simulink model "linModel_S_LQG"  (R2021b)
settings: Solver=ode45  StartTime=0.0  StopTime=0.5  MaxStep=0.01  RelTol=1e-8
values from neighbouring files (symbols this model uses):
  A = [0 1; -k/mass-(4*C_magnetic*Ib^2)/(mass*gap^3) -c/mass]    [ex4.m]    (also in mp62.m = [-2 -3;-1 -4]; od.m = [0 1; -k/m-(4*C_magnetic*Ib^2)/(m*gap^3) -c/m])
  B = [0;(4*C_magnetic*Ib)/(mass*gap^2)]    [ex4.m]    (also in mp62.m = [0 1]'; od.m = [0;(4*C_magnetic*Ib)/(m*gap^2)])
  C = 0.0157    [ex2_1.m]    (also in ex3.m = 3.73e-06; ex4.m = [1 0]; mp62.m = [1 0]; od.m = [1 0;0 0])
  D = 0    [ex4.m]    (also in mp62.m; od.m)
  Kf = lqr(A',C',Vd,Vn)    [ex4.m]
  L = acker(A',C',P)'    [mp62.m]
undefined symbols (not defined in the file or in its folder): Kr
settings Model: Creator=danli  LastModifiedBy=danli

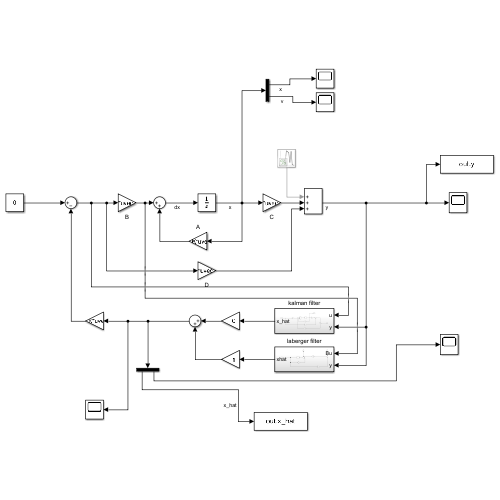
[thumbnail: Simulink's stored preview of the top-level diagram]
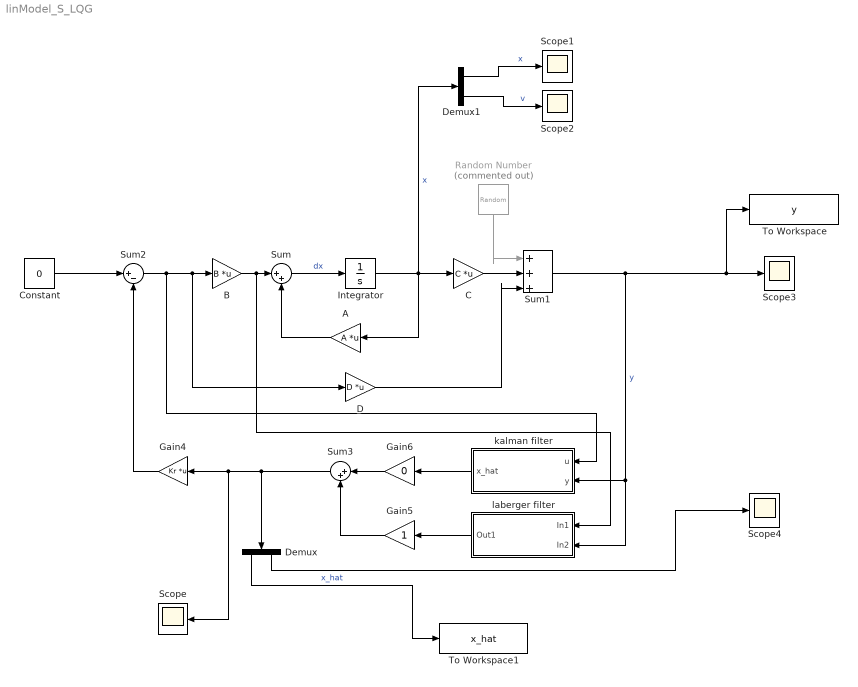
== system linModel_S_LQG ==
  A : Gain  Gain=A  Multiplication=Matrix(K*u) (u vector)
  B : Gain  Gain=B  Multiplication=Matrix(K*u) (u vector)
  C : Gain  Gain=C  Multiplication=Matrix(K*u) (u vector)
  Constant : Constant  Value=0
  D : Gain  Gain=D  Multiplication=Matrix(K*u) (u vector)
  Demux : Demux  Outputs=2
  Demux1 : Demux  Outputs=2
  Gain4 : Gain  Gain=Kr  Multiplication=Matrix(K*u) (u vector)
  Gain5 : Gain
  Gain6 : Gain  Gain=0
  Integrator : Integrator  InitialCondition=[5*10^-5 0]
  Random Number : RandomNumber  Commented=on  Variance=0.0000000000001  SampleTime=0.001
  Scope{,1..4} (5 alike) : Scope
  Sum : Sum  Inputs=|++
  Sum1 : Sum  Inputs=|+|+|+
  Sum2 : Sum  Inputs=|+-
  Sum3 : Sum  Inputs=|++
  To Workspace : ToWorkspace  VariableName=y  SaveFormat=Timeseries  SampleTime=-1
  To Workspace1 : ToWorkspace  VariableName=x_hat  SaveFormat=Timeseries  SampleTime=-1
  kalman filter : Subsystem
  laberger filter : Subsystem
  wires:
  B/1 -> laberger filter/1(In1), Sum/1
  A/1 -> Sum/2
  Sum/1 -> Integrator/1  "dx"
  Integrator/1 -> A/1, Demux1/1, C/1  "x"
  D/1 -> Sum1/3
  C/1 -> Sum1/2
  Sum2/1 -> kalman filter/1(u), D/1, B/1
  Constant/1 -> Sum2/1
  Gain4/1 -> Sum2/2
  Demux1/1 -> Scope1/1  "x"
  Demux1/2 -> Scope2/1  "v"
  Sum1/1 -> To Workspace/1, Scope3/1, laberger filter/2(In2), kalman filter/2(y)  "y"
  Random Number/1 -> Sum1/1
  Demux/1 -> To Workspace1/1  "x_hat"
  Demux/2 -> Scope4/1
  laberger filter/1(Out1) -> Gain5/1
  Gain5/1 -> Sum3/2
  kalman filter/1(x_hat) -> Gain6/1
  Gain6/1 -> Sum3/1
  Sum3/1 -> Demux/1, Scope/1, Gain4/1

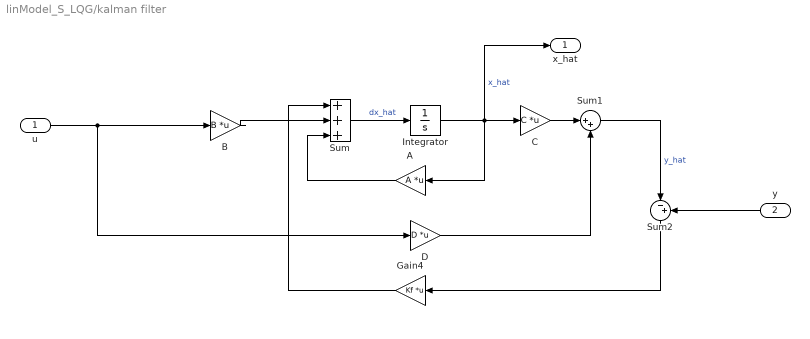
== system linModel_S_LQG/kalman filter ==
  u : Inport
  y : Inport  Port=2
  A : Gain  Gain=A  Multiplication=Matrix(K*u) (u vector)
  B : Gain  Gain=B  Multiplication=Matrix(K*u) (u vector)
  C : Gain  Gain=C  Multiplication=Matrix(K*u) (u vector)
  D : Gain  Gain=D  Multiplication=Matrix(K*u) (u vector)
  Gain4 : Gain  Gain=Kf  Multiplication=Matrix(K*u) (u vector)
  Integrator : Integrator  InitialCondition=[3*10^-5 0]
  Sum : Sum  Inputs=|+++
  Sum1 : Sum  Inputs=|++
  Sum2 : Sum  Inputs=|-+
  x_hat : Outport
  wires:
  Sum1/1 -> Sum2/1  "y_hat"
  Integrator/1 -> x_hat/1, A/1, C/1  "x_hat"
  D/1 -> Sum1/2
  C/1 -> Sum1/1
  Sum/1 -> Integrator/1  "dx_hat"
  A/1 -> Sum/3
  y/1 -> Sum2/2
  Sum2/1 -> Gain4/1
  Gain4/1 -> Sum/1
  u/1 -> B/1, D/1
  B/1 -> Sum/2

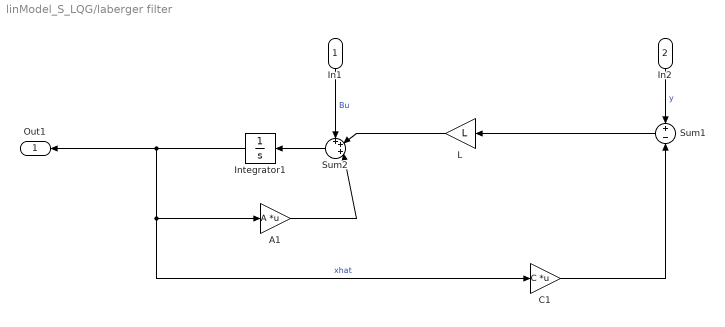
== system linModel_S_LQG/laberger filter ==
  In1 : Inport
  In2 : Inport  Port=2
  A1 : Gain  Gain=A  Multiplication=Matrix(K*u) (u vector)
  C1 : Gain  Gain=C  Multiplication=Matrix(K*u) (u vector)
  Integrator1 : Integrator  InitialCondition=[3*10^-5 0]'
  L : Gain  Gain=L
  Sum1 : Sum  Inputs=+|-
  Sum2 : Sum  Inputs=+++|
  Out1 : Outport
  wires:
  Integrator1/1 -> C1/1, A1/1, Out1/1  "xhat"
  In1/1 -> Sum2/1  "Bu"
  Sum1/1 -> L/1
  A1/1 -> Sum2/3
  In2/1 -> Sum1/1  "y"
  Sum2/1 -> Integrator1/1
  L/1 -> Sum2/2
  C1/1 -> Sum1/2
